simulink model "PFChysterisiscontrol"  (R2020a)
settings: Solver=ode8  StartTime=0.0  StopTime=0.8  FixedStep=1e-5  RelTol=1e-3
libraries: powerlib x16, powerlib_meascontrol x3, simulink x1
settings Model: Creator=ASUS User  LastModifiedBy=Mayouch
settings SolverCC: ZeroCrossAlgorithm=Adaptive
settings DataIOCC: ReturnWorkspaceOutputs=off
settings DebuggingCC: MaxConsecutiveZCsMsg=none  ArithmeticOperatorsInVariantConditions=warning
settings SFSimCC: SimUseLocalCustomCode=off  CustomCodeUndefinedFunction=UseInterfaceOnly
settings RTWCC: RTWUseLocalCustomCode=off

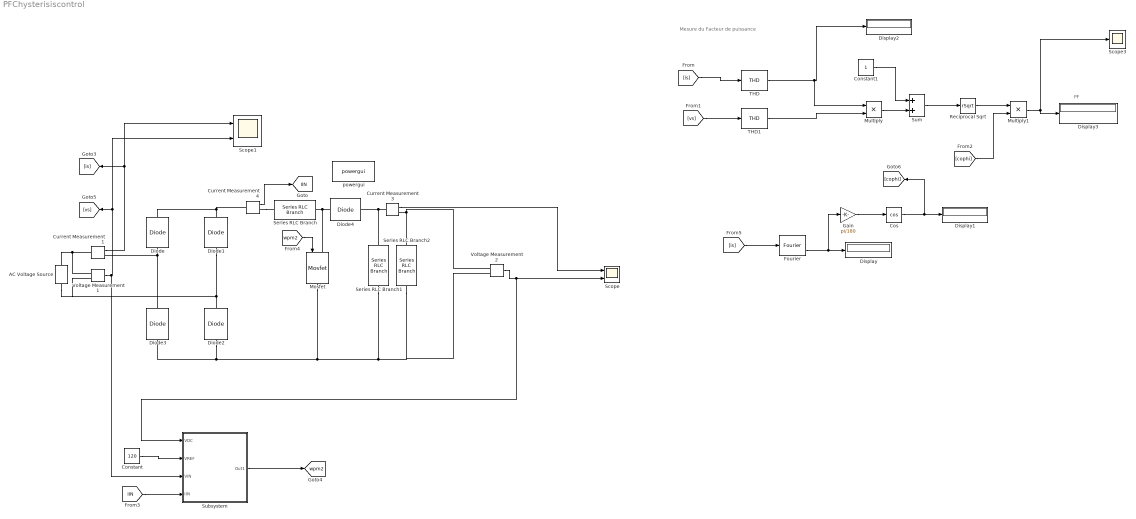
== system PFChysterisiscontrol ==
  note: Mesure du Facteur de puissance
  note: PF
  AC Voltage Source : powerlib/Electrical Sources/AC Voltage Source  Amplitude=60*sqrt(2)  Phase=0  Frequency=50  SampleTime=0  Measurements=None  BusType=swing  Pref=10e3  Qref=0  Qmin=-inf  Qmax=+inf
  Constant : Constant  Value=120
  Constant1 : Constant
  Cos : Trigonometry  Operator=cos
  Current Measurement1 : powerlib/Measurements/Current Measurement  PhasorSimulation=off  OutputType=Complex  PSBequivalent=0
  Current Measurement3 : powerlib/Measurements/Current Measurement  PhasorSimulation=off  OutputType=Complex  PSBequivalent=0
  Current Measurement4 : powerlib/Measurements/Current Measurement  PhasorSimulation=off  OutputType=Complex  PSBequivalent=0
  Diode{,1..4} (5 alike) : powerlib/Power Electronics/Diode  Ron=0.001  Lon=0  Vf=0.8  IC=0  UseSnubber=0  Rs=500  Cs=250e-9  Measurements=off
  Display{,1..3} (4 alike) : Display
  Fourier : powerlib_meascontrol/Measurements/Fourier  Freq=50  n=1  InInit=[0, 0]  Ts=0
  Gain : Gain  Gain=pi/180
  Mosfet : powerlib/Power Electronics/Mosfet  Ron=0.1  Lon=0  Rd=0.01  Vfd=0  IC=0  Rs=1e5  Cs=inf  Measurements=off
  Multiply : Product
  Multiply1 : Product
  Reciprocal Sqrt : Sqrt  Operator=rSqrt  SaturateOnIntegerOverflow=on
  Scope : Scope  NumInputPorts=2
  Scope1 : Scope  NumInputPorts=2
  Scope3 : Scope
  Series RLC Branch : powerlib/Elements/Series RLC Branch  LConnTagsString=__new0  RConnTagsString=__new0  BranchType=L  Resistance=1  Inductance=9.5e-3  SetiL0=off  InitialCurrent=0  Capacitance=1e-6  Setx0=off  InitialVoltage=0  Measurements=None
  Series RLC Branch1 : powerlib/Elements/Series RLC Branch  LConnTagsString=__new0  RConnTagsString=__new0  BranchType=C  Resistance=1  Inductance=1e-3  SetiL0=off  InitialCurrent=0  Capacitance=2200e-6  Setx0=off  InitialVoltage=100  Measurements=None
  Series RLC Branch2 : powerlib/Elements/Series RLC Branch  LConnTagsString=__new0  RConnTagsString=__new0  BranchType=R  Resistance=90  Inductance=1e-3  SetiL0=off  InitialCurrent=0  Capacitance=1e-6  Setx0=off  InitialVoltage=0  Measurements=None
  Subsystem : Subsystem
  Sum : Sum
  THD : powerlib_meascontrol/Measurements/THD  Freq=50  Ts=0
  THD1 : powerlib_meascontrol/Measurements/THD  Freq=50  Ts=0
  Voltage Measurement1 : powerlib/Measurements/Voltage Measurement  PhasorSimulation=off  OutputType=Complex  PSBequivalent=0
  Voltage Measurement2 : powerlib/Measurements/Voltage Measurement  PhasorSimulation=off  OutputType=Complex  PSBequivalent=0
  powergui : powerlib/powergui  Priority=1  SimulationMode=Discrete  SampleTime=1e-5  frequency=60  Iterations=50  frequencyindice=50  Pbase=100e6  ErrMax=1e-4  UnitsV=kV  UnitsW=MW  buscounter=0  FunctionMessages=off  echomessages=off  EnableUseOfTLC=off  CurrentSourceSwitches=off  DisableSnubberDevices=off  DisableRonSwitches=off  DisableVfSwitches=off  DisplayEquations=off  AutomaticDiscreteSolvers=off  SolverType=Tustin/Backward Euler (TBE)  Interpol=off  ExternalGateDelay=off  methode=off  Ts=100  x0status=blocks  SPID=off  SwTol=0  HookPort=off  NonlinearTolerance=1e-4  nMaxIteration=100  ContinueOnMaxIteration=off  RestoreLinks=warning  ResistiveCurrentMeasurement=off  Frange=[0:2:500]  Ylog=off  Xlog=on  ShowGrid=off  save=off  variable=ZData  structure=ScopeData1  ZoomFFT=on  StartTime=0.1  cycles=5  DisplayStyle=1  fundamental=50  FreqAxis=on  MaxFrequency=500  frequencyindicesteady=1  RmsSteady=1  display=off
  tag scope: IIN=global, wpm2=global
  wires:
  Voltage Measurement1/1 -> Scope1/2, [vs], Subsystem/3(VIN)
  Constant/1 -> Subsystem/2(VREF)
  Current Measurement3/1 -> Scope/1
  Current Measurement1/1 -> Scope1/1, [is]
  Fourier/2 -> Gain/1, Display/1
  Gain/1 -> Cos/1
  Voltage Measurement2/1 -> Subsystem/1(VDC), Scope/2
  Subsystem/1(Out1) -> [wpm2]
  [wpm2] -> Mosfet/1
  THD/1 -> Multiply/1, Display2/1
  [vs] -> THD1/1
  [is] -> THD/1
  THD1/1 -> Multiply/2
  Multiply/1 -> Sum/2
  Constant1/1 -> Sum/1
  Sum/1 -> Reciprocal Sqrt/1
  Reciprocal Sqrt/1 -> Multiply1/1
  Cos/1 -> [cophi], Display1/1
  [cophi] -> Multiply1/2
  Multiply1/1 -> Scope3/1, Display3/1
  [is] -> Fourier/1
  Current Measurement4/1 -> [IIN]
  [IIN] -> Subsystem/4(IIN)
  connections:
  Diode/LConn1 -- Current Measurement1/RConn1 -- Diode3/RConn1
  Diode1/LConn1 -- Voltage Measurement1/LConn2 -- AC Voltage Source/LConn1 -- Diode2/RConn1
  Diode2/LConn1 -- Voltage Measurement2/LConn2 -- Series RLC Branch2/RConn1 -- Series RLC Branch1/RConn1 -- Mosfet/RConn1 -- Diode3/LConn1
  Diode/RConn1 -- Current Measurement4/LConn1 -- Diode1/RConn1
  Series RLC Branch/RConn1 -- Diode4/LConn1 -- Mosfet/LConn1
  Series RLC Branch1/LConn1 -- Current Measurement3/LConn1 -- Diode4/RConn1
  AC Voltage Source/RConn1 -- Voltage Measurement1/LConn1 -- Current Measurement1/LConn1
  Current Measurement4/RConn1 -- Series RLC Branch/LConn1
  Current Measurement3/RConn1 -- Voltage Measurement2/LConn1 -- Series RLC Branch2/LConn1

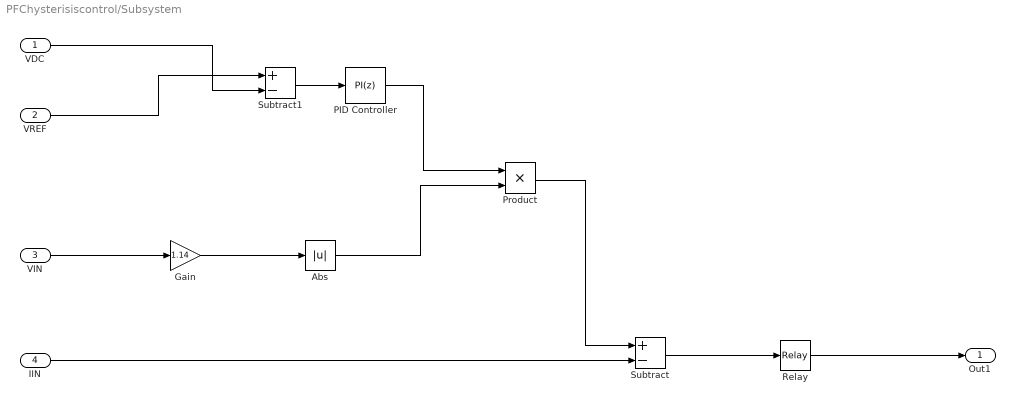
== system PFChysterisiscontrol/Subsystem ==
  VDC : Inport
  VREF : Inport  Port=2
  VIN : Inport  Port=3
  IIN : Inport  Port=4
  Abs : Abs
  Gain : Gain  Gain=1.14
  PID Controller : simulink/Continuous/PID Controller  Controller=PI  Form=Parallel  TimeDomain=Discrete-time  UseExternalTs=off  SampleTime=-1  IntegratorMethod=Forward Euler  FilterMethod=Forward Euler  ControllerParametersSource=internal  P=0.00200832981814989  I=0.0513084230123843  D=0  UseFilter=on  N=100  TunerSelectOption=Transfer Function Based (PID Tuner App)  InitialConditionSource=internal  InitialConditionForIntegrator=0  InitialConditionForFilter=0  DifferentiatorICPrevScaledInput=0  ExternalReset=none  TrackingMode=off  Kt=1  LimitOutput=off  UpperSaturationLimit=0.1  LowerSaturationLimit=0  LinearizeAsGain=on  AntiWindupMode=none  Kb=1  POutMin=[]  POutMax=[]  IOutMin=[]  IOutMax=[]  DOutMin=[]  DOutMax=[]  NOutMin=[]  NOutMax=[]  SumOutMin=[]  SumOutMax=[]  SaturationOutMin=[]  SaturationOutMax=[]  PParamMin=[]  PParamMax=[]  IParamMin=[]  IParamMax=[]  DParamMin=[]  DParamMax=[]  NParamMin=[]  NParamMax=[]  KbParamMin=[]  KbParamMax=[]  KtParamMin=[]  KtParamMax=[]  KbOutMin=[]  KbOutMax=[]  KtOutMin=[]  KtOutMax=[]  IntegratorOutMin=[]  IntegratorOutMax=[]  FilterOutMin=[]  FilterOutMax=[]  SumI1OutMin=[]  SumI1OutMax=[]  SumI2OutMin=[]  SumI2OutMax=[]  SumI3OutMin=[]  SumI3OutMax=[]  SumI4OutMin=[]  SumI4OutMax=[]  SumDOutMin=[]  SumDOutMax=[]  DifferentiatorOutMin=[]  DifferentiatorOutMax=[]  FilterDiffOutCoefMin=[]  FilterDiffOutCoefMax=[]  ReciprocalOutMin=[]  ReciprocalOutMax=[]  SumDenOutMin=[]  SumDenOutMax=[]  SumNumOutMin=[]  SumNumOutMax=[]  DivideOutMin=[]  DivideOutMax=[]  UdiffTsProdOutMin=[]  UdiffTsProdOutMax=[]  NTsProdOutMin=[]  NTsProdOutMax=[]  UintegralTsProdOutMin=[]  UintegralTsProdOutMax=[]  UngainTsProdOutMin=[]  UngainTsProdOutMax=[]  IntegratorContinuousStateAttributes=''  IntegratorStateMustResolveToSignalObject=off  IntegratorRTWStateStorageClass=Auto  FilterContinuousStateAttributes=''  FilterStateMustResolveToSignalObject=off  FilterRTWStateStorageClass=Auto  ParallelPVariant=InternalParameters  IdealPVariant=Disabled  IVariant=InternalParameters  DVariant=Disabled  IntegratorVariant=Discrete  SatVariant=Disabled  AWVariant=Passthrough  PCopyVariant=Disabled  TRVariant=Disabled  FdbkBlocksVariant=Forward  IdealPFdbkVariant=Disabled  SatFdbkVariant=Disabled  DerivativeFilterVariant=Disabled  NVariant=Disabled  NCopyVariant=Disabled_SignalSpec  FilterICVariant=Disabled  IntegratorICVariant=InternalICs  ExternalResetVariant=Disabled  TRSumVariant=Passthrough  SumFdbkVariant=Disabled  SumVariant=Sum_PI  TsampFilterVariant=InternalTs  TsampNgainVariant=Passthrough  TsampIntegralVariant=Passthrough
  Product : Product
  Relay : Relay  OnSwitchValue=0.001  OffSwitchValue=-0.001
  Subtract : Sum  Inputs=+-
  Subtract1 : Sum  Inputs=+-
  Out1 : Outport  VectorParamsAs1DForOutWhenUnconnected=off
  wires:
  PID Controller/1 -> Product/1
  VREF/1 -> Subtract1/1
  Abs/1 -> Product/2
  Product/1 -> Subtract/1
  VDC/1 -> Subtract1/2
  IIN/1 -> Subtract/2
  Subtract/1 -> Relay/1
  Gain/1 -> Abs/1
  VIN/1 -> Gain/1
  Subtract1/1 -> PID Controller/1
  Relay/1 -> Out1/1
